simulink model "tres_tt_threeservos"  (Simulink 8.3)
settings: Solver=ode45  StartTime=0.0  StopTime=1.0  RelTol=1e-3
libraries: tres_simulink_blockset x4, truetime x1
settings Model: Creator=matteo  LastModifiedBy=matteo
settings OptimizationCC: ExpressionDepthLimit=2147483647
settings DebuggingCC: FcnCallInpInsideContextMsg=EnableAllAsWarning
settings GRTTargetCC: CombineOutputUpdateFcns=on  GRTInterface=off

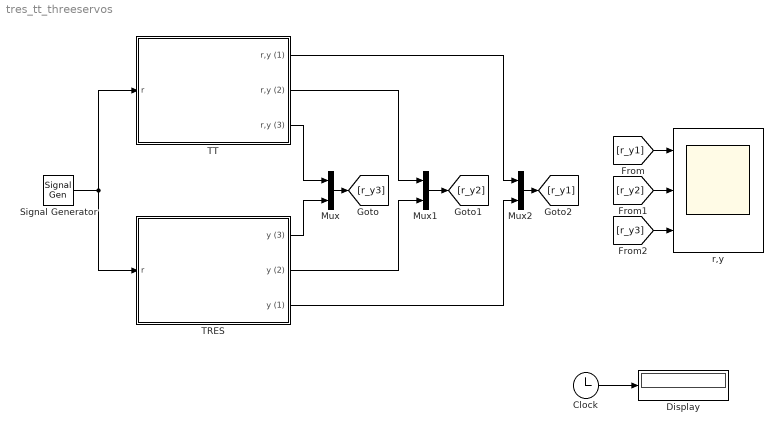
== system tres_tt_threeservos ==
  Clock : Clock
  Display : Display
  Mux : Mux  Inputs=2
  Mux1 : Mux  Inputs=2
  Mux2 : Mux  Inputs=2
  Signal Generator : SignalGenerator  WaveForm=square  Frequency=1.5
  TRES : Subsystem  TreatAsAtomicUnit=on
  TT : Subsystem  TreatAsAtomicUnit=on
  r,y : Scope  NumInputPorts=3
      settings: TimeRange=1  YMin=-2~-2~-2  YMax=2~2~2  SaveName=ry
  wires:
  Clock/1 -> Display/1
  TT/3(r,y (3)) -> Mux/1
  TRES/1(y (3)) -> Mux/2
  TRES/2(y (2)) -> Mux1/2
  TT/2(r,y (2)) -> Mux1/1
  TRES/3(y (1)) -> Mux2/2
  TT/1(r,y (1)) -> Mux2/1
  Mux/1 -> [r_y3]
  Mux1/1 -> [r_y2]
  Mux2/1 -> [r_y1]
  [r_y1] -> r,y/1
  [r_y2] -> r,y/2
  [r_y3] -> r,y/3
  Signal Generator/1 -> TT/1(r), TRES/1(r)

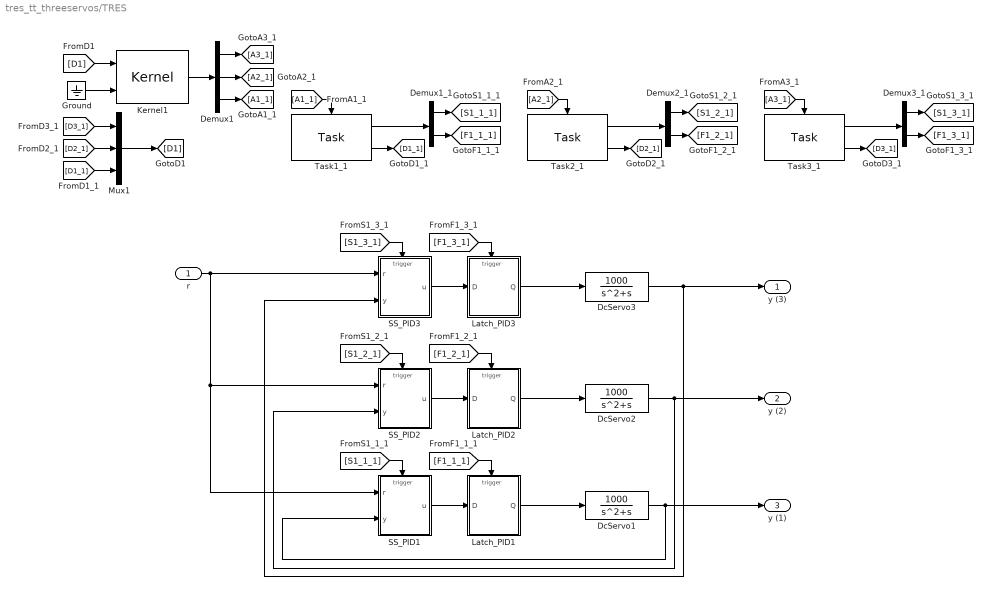
== system tres_tt_threeservos/TRES ==
  r : Inport
  DcServo1 : TransferFcn  Numerator=[1000]  Denominator=[1 1 0]
  DcServo2 : TransferFcn  Numerator=[1000]  Denominator=[1 1 0]
  DcServo3 : TransferFcn  Numerator=[1000]  Denominator=[1 1 0]
  Demux1 : Demux  Outputs=3
  Demux1_1 : Demux  Outputs=2
  Demux2_1 : Demux  Outputs=2
  Demux3_1 : Demux  Outputs=2
  Ground : Ground
  Kernel1 : tres_simulink_blockset/Kernel  taskset_descr_name=task_set_descr  scheduling_policy=DEADLINE_MONOTONIC  dead_miss_rule=Continue  time_res=Milli_Seconds  core_num=1  under_engine=RTSIM
  Latch_PID1 : Subsystem  TreatAsAtomicUnit=on
  Latch_PID2 : Subsystem  TreatAsAtomicUnit=on
  Latch_PID3 : Subsystem  TreatAsAtomicUnit=on
  Mux1 : Mux  Inputs=3
  SS_PID1 : Subsystem
  SS_PID2 : Subsystem
  SS_PID3 : Subsystem
  Task1_1 : tres_simulink_blockset/Task  conf_name=task1_1_descr
  Task2_1 : tres_simulink_blockset/Task  conf_name=task2_1_descr
  Task3_1 : tres_simulink_blockset/Task  conf_name=task3_1_descr
  y (3) : Outport
  y (2) : Outport  Port=2
  y (1) : Outport  Port=3
  wires:
  r/1 -> SS_PID1/1(r), SS_PID2/1(r), SS_PID3/1(r)
  DcServo3/1 -> SS_PID3/2(y), y (3)/1
  DcServo2/1 -> SS_PID2/2(y), y (2)/1
  DcServo1/1 -> SS_PID1/2(y), y (1)/1
  SS_PID3/1(u) -> Latch_PID3/1(D)
  SS_PID2/1(u) -> Latch_PID2/1(D)
  SS_PID1/1(u) -> Latch_PID1/1(D)
  Kernel1/1 -> Demux1/1
  Demux1/1 -> [A3_1]
  [D3_1] -> Mux1/1
  Demux1/2 -> [A2_1]
  [D2_1] -> Mux1/2
  Demux1/3 -> [A1_1]
  [D1_1] -> Mux1/3
  [D1] -> Kernel1/1
  Mux1/1 -> [D1]
  Task1_1/2 -> [D1_1]
  [A1_1] -> Task1_1/Trigger
  Task1_1/1 -> Demux1_1/1
  Demux1_1/1 -> [S1_1_1]
  Demux1_1/2 -> [F1_1_1]
  Task2_1/2 -> [D2_1]
  [A2_1] -> Task2_1/Trigger
  Task2_1/1 -> Demux2_1/1
  Demux2_1/1 -> [S1_2_1]
  Demux2_1/2 -> [F1_2_1]
  Task3_1/2 -> [D3_1]
  [A3_1] -> Task3_1/Trigger
  Task3_1/1 -> Demux3_1/1
  Demux3_1/1 -> [S1_3_1]
  Demux3_1/2 -> [F1_3_1]
  Latch_PID1/1(Q) -> DcServo1/1
  [S1_1_1] -> SS_PID1/Trigger
  [F1_1_1] -> Latch_PID1/Trigger
  Latch_PID2/1(Q) -> DcServo2/1
  [S1_2_1] -> SS_PID2/Trigger
  [F1_2_1] -> Latch_PID2/Trigger
  Latch_PID3/1(Q) -> DcServo3/1
  [S1_3_1] -> SS_PID3/Trigger
  [F1_3_1] -> Latch_PID3/Trigger
  Ground/1 -> Kernel1/2

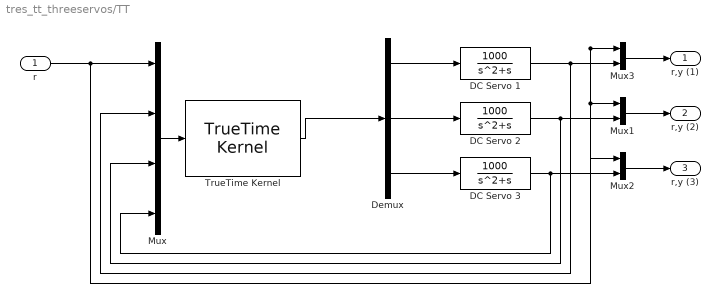
== system tres_tt_threeservos/TT ==
  r : Inport
  DC Servo 1 : TransferFcn  Numerator=[1000]  Denominator=[1 1 0]
  DC Servo 2 : TransferFcn  Numerator=[1000]  Denominator=[1 1 0]
  DC Servo 3 : TransferFcn  Numerator=[1000]  Denominator=[1 1 0]
  Demux : Demux  Outputs=3
  Mux : Mux
  Mux1 : Mux  Inputs=2
  Mux2 : Mux  Inputs=2
  Mux3 : Mux  Inputs=2
  TrueTime Kernel : truetime/TrueTime Kernel  sfun=tt_threeservos_init  args=1  ninputsoutputs=[4 3]  ntriggers=0  trigtype=falling  nwnodenbr=[]  clockoffsetdrift=[0 0]  schedoutput=off  battery=off  poweroutput=off
  r,y (1) : Outport
  r,y (2) : Outport  Port=2
  r,y (3) : Outport  Port=3
  wires:
  r/1 -> Mux1/1, Mux2/1, Mux3/1, Mux/1
  Demux/2 -> DC Servo 2/1
  Demux/3 -> DC Servo 3/1
  DC Servo 1/1 -> Mux3/2, Mux/2
  DC Servo 2/1 -> Mux1/2, Mux/3
  DC Servo 3/1 -> Mux2/2, Mux/4
  Mux2/1 -> r,y (3)/1
  Mux/1 -> TrueTime Kernel/1
  TrueTime Kernel/1 -> Demux/1
  Mux1/1 -> r,y (2)/1
  Mux3/1 -> r,y (1)/1
  Demux/1 -> DC Servo 1/1

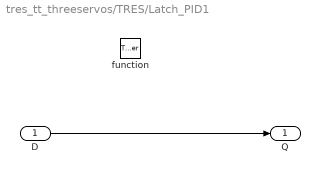
== system tres_tt_threeservos/TRES/Latch_PID1 ==
  D : Inport
  function : TriggerPort  TriggerType=function-call
  Q : Outport
  wires:
  D/1 -> Q/1

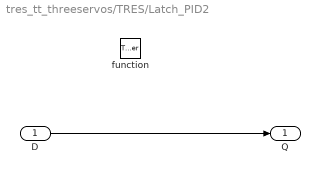
== system tres_tt_threeservos/TRES/Latch_PID2 ==
  D : Inport
  function : TriggerPort  TriggerType=function-call
  Q : Outport
  wires:
  D/1 -> Q/1

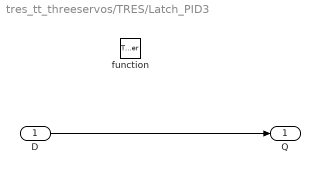
== system tres_tt_threeservos/TRES/Latch_PID3 ==
  D : Inport
  function : TriggerPort  TriggerType=function-call
  Q : Outport
  wires:
  D/1 -> Q/1

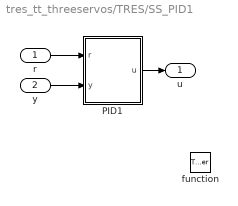
== system tres_tt_threeservos/TRES/SS_PID1 ==
  r : Inport
  y : Inport  Port=2
  function : TriggerPort  TriggerType=function-call
  PID1 : Subsystem  mask{K=0.96, Ti=0.12, Td=0.049, beta=0.5, N=10, h=0.006}
  u : Outport
  wires:
  r/1 -> PID1/1(r)
  y/1 -> PID1/2(y)
  PID1/1(u) -> u/1

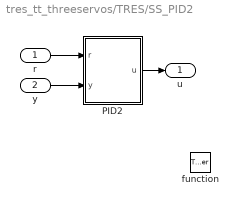
== system tres_tt_threeservos/TRES/SS_PID2 ==
  r : Inport
  y : Inport  Port=2
  function : TriggerPort  TriggerType=function-call
  PID2 : Subsystem  mask{K=0.96, Ti=0.12, Td=0.049, beta=0.5, N=10, h=0.005}
  u : Outport
  wires:
  r/1 -> PID2/1(r)
  y/1 -> PID2/2(y)
  PID2/1(u) -> u/1

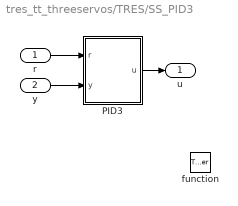
== system tres_tt_threeservos/TRES/SS_PID3 ==
  r : Inport
  y : Inport  Port=2
  function : TriggerPort  TriggerType=function-call
  PID3 : Subsystem  mask{K=0.96, Ti=0.12, Td=0.049, beta=0.5, N=10, h=0.004}
  u : Outport
  wires:
  r/1 -> PID3/1(r)
  y/1 -> PID3/2(y)
  PID3/1(u) -> u/1

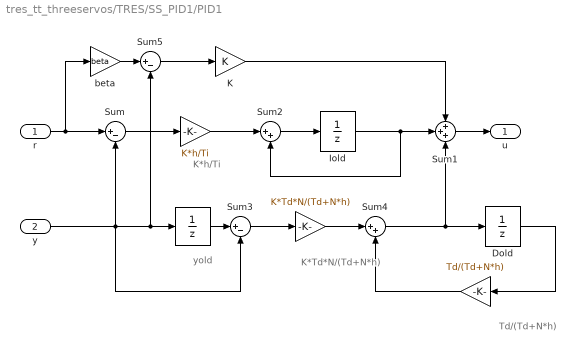
== system tres_tt_threeservos/TRES/SS_PID1/PID1 ==
  note: K*h/Ti
  note: K*Td*N/(Td+N*h)
  note: Td/(Td+N*h)
  note: yold
  r : Inport  SampleTime=-1.0
  y : Inport  Port=2  SampleTime=-1.0
  " " : UnitDelay  SampleTime=-1.0
  "   " : Gain  Gain=K*h/Ti  SampleTime=-1.0  SaturateOnIntegerOverflow=on  OutDataTypeStr=Inherit: Same as input  ParamDataTypeStr=Inherit: Same as input
  "             " : Gain  Gain=K*Td*N/(Td+N*h)  SampleTime=-1.0  SaturateOnIntegerOverflow=on  OutDataTypeStr=Inherit: Same as input  ParamDataTypeStr=Inherit: Same as input
  "              " : Gain  Gain=Td/(Td+N*h)  SampleTime=-1.0  SaturateOnIntegerOverflow=on  OutDataTypeStr=Inherit: Same as input  ParamDataTypeStr=Inherit: Same as input
  Dold : UnitDelay  SampleTime=-1.0
  "Iold " : UnitDelay  SampleTime=-1.0
  K : Gain  Gain=K  SampleTime=-1.0  SaturateOnIntegerOverflow=on  OutDataTypeStr=Inherit: Same as input  ParamDataTypeStr=Inherit: Same as input
  Sum : Sum  Inputs=|+-  SampleTime=-1.0  SaturateOnIntegerOverflow=on  InputSameDT=on  OutDataTypeStr=Inherit: Same as first input
  Sum1 : Sum  Inputs=+++  SampleTime=-1.0  SaturateOnIntegerOverflow=on  InputSameDT=on  OutDataTypeStr=Inherit: Same as first input
  Sum2 : Sum  Inputs=|++  SampleTime=-1.0  SaturateOnIntegerOverflow=on  InputSameDT=on  OutDataTypeStr=Inherit: Same as first input
  Sum3 : Sum  Inputs=|+-  SampleTime=-1.0  SaturateOnIntegerOverflow=on  InputSameDT=on  OutDataTypeStr=Inherit: Same as first input
  Sum4 : Sum  Inputs=|++  SampleTime=-1.0  SaturateOnIntegerOverflow=on  InputSameDT=on  OutDataTypeStr=Inherit: Same as first input
  Sum5 : Sum  Inputs=|+-  SampleTime=-1.0  SaturateOnIntegerOverflow=on  InputSameDT=on  OutDataTypeStr=Inherit: Same as first input
  beta : Gain  Gain=beta  SampleTime=-1.0  SaturateOnIntegerOverflow=on  OutDataTypeStr=Inherit: Same as input  ParamDataTypeStr=Inherit: Same as input
  u : Outport  SampleTime=-1.0
  wires:
  y/1 -> Sum/2, Sum3/2, " "/1, Sum5/2
  r/1 -> Sum/1, beta/1
  Sum1/1 -> u/1
  K/1 -> Sum1/1
  Sum2/1 -> "Iold "/1
  Dold/1 -> "              "/1
  "             "/1 -> Sum4/1
  Sum3/1 -> "             "/1
  Sum4/1 -> Dold/1, Sum1/3
  " "/1 -> Sum3/1
  "Iold "/1 -> Sum2/2, Sum1/2
  "   "/1 -> Sum2/1
  Sum/1 -> "   "/1
  "              "/1 -> Sum4/2
  beta/1 -> Sum5/1
  Sum5/1 -> K/1

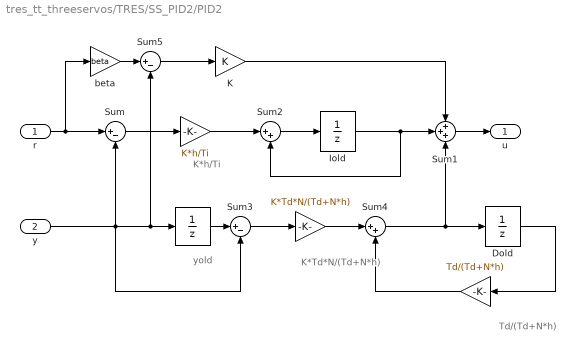
== system tres_tt_threeservos/TRES/SS_PID2/PID2 ==
  note: K*h/Ti
  note: K*Td*N/(Td+N*h)
  note: Td/(Td+N*h)
  note: yold
  r : Inport  SampleTime=-1.0
  y : Inport  Port=2  SampleTime=-1.0
  " " : UnitDelay  SampleTime=-1.0
  "   " : Gain  Gain=K*h/Ti  SampleTime=-1.0  SaturateOnIntegerOverflow=on  OutDataTypeStr=Inherit: Same as input  ParamDataTypeStr=Inherit: Same as input
  "             " : Gain  Gain=K*Td*N/(Td+N*h)  SampleTime=-1.0  SaturateOnIntegerOverflow=on  OutDataTypeStr=Inherit: Same as input  ParamDataTypeStr=Inherit: Same as input
  "              " : Gain  Gain=Td/(Td+N*h)  SampleTime=-1.0  SaturateOnIntegerOverflow=on  OutDataTypeStr=Inherit: Same as input  ParamDataTypeStr=Inherit: Same as input
  Dold : UnitDelay  SampleTime=-1.0
  "Iold " : UnitDelay  SampleTime=-1.0
  K : Gain  Gain=K  SampleTime=-1.0  SaturateOnIntegerOverflow=on  OutDataTypeStr=Inherit: Same as input  ParamDataTypeStr=Inherit: Same as input
  Sum : Sum  Inputs=|+-  SampleTime=-1.0  SaturateOnIntegerOverflow=on  InputSameDT=on  OutDataTypeStr=Inherit: Same as first input
  Sum1 : Sum  Inputs=+++  SampleTime=-1.0  SaturateOnIntegerOverflow=on  InputSameDT=on  OutDataTypeStr=Inherit: Same as first input
  Sum2 : Sum  Inputs=|++  SampleTime=-1.0  SaturateOnIntegerOverflow=on  InputSameDT=on  OutDataTypeStr=Inherit: Same as first input
  Sum3 : Sum  Inputs=|+-  SampleTime=-1.0  SaturateOnIntegerOverflow=on  InputSameDT=on  OutDataTypeStr=Inherit: Same as first input
  Sum4 : Sum  Inputs=|++  SampleTime=-1.0  SaturateOnIntegerOverflow=on  InputSameDT=on  OutDataTypeStr=Inherit: Same as first input
  Sum5 : Sum  Inputs=|+-  SampleTime=-1.0  SaturateOnIntegerOverflow=on  InputSameDT=on  OutDataTypeStr=Inherit: Same as first input
  beta : Gain  Gain=beta  SampleTime=-1.0  SaturateOnIntegerOverflow=on  OutDataTypeStr=Inherit: Same as input  ParamDataTypeStr=Inherit: Same as input
  u : Outport  SampleTime=-1.0
  wires:
  y/1 -> Sum/2, Sum3/2, " "/1, Sum5/2
  r/1 -> Sum/1, beta/1
  Sum1/1 -> u/1
  K/1 -> Sum1/1
  Sum2/1 -> "Iold "/1
  Dold/1 -> "              "/1
  "             "/1 -> Sum4/1
  Sum3/1 -> "             "/1
  Sum4/1 -> Dold/1, Sum1/3
  " "/1 -> Sum3/1
  "Iold "/1 -> Sum2/2, Sum1/2
  "   "/1 -> Sum2/1
  Sum/1 -> "   "/1
  "              "/1 -> Sum4/2
  beta/1 -> Sum5/1
  Sum5/1 -> K/1

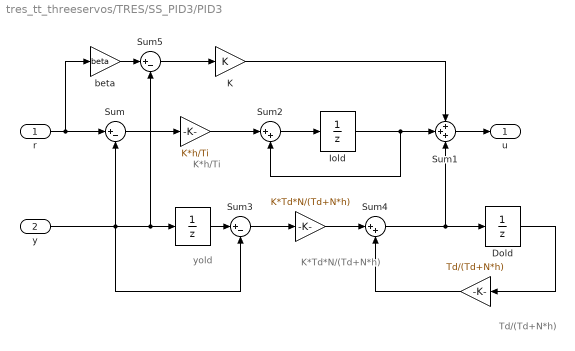
== system tres_tt_threeservos/TRES/SS_PID3/PID3 ==
  note: K*h/Ti
  note: K*Td*N/(Td+N*h)
  note: Td/(Td+N*h)
  note: yold
  r : Inport  SampleTime=-1.0
  y : Inport  Port=2  SampleTime=-1.0
  " " : UnitDelay  SampleTime=-1.0
  "   " : Gain  Gain=K*h/Ti  SampleTime=-1.0  SaturateOnIntegerOverflow=on  OutDataTypeStr=Inherit: Same as input  ParamDataTypeStr=Inherit: Same as input
  "             " : Gain  Gain=K*Td*N/(Td+N*h)  SampleTime=-1.0  SaturateOnIntegerOverflow=on  OutDataTypeStr=Inherit: Same as input  ParamDataTypeStr=Inherit: Same as input
  "              " : Gain  Gain=Td/(Td+N*h)  SampleTime=-1.0  SaturateOnIntegerOverflow=on  OutDataTypeStr=Inherit: Same as input  ParamDataTypeStr=Inherit: Same as input
  Dold : UnitDelay  SampleTime=-1.0
  "Iold " : UnitDelay  SampleTime=-1.0
  K : Gain  Gain=K  SampleTime=-1.0  SaturateOnIntegerOverflow=on  OutDataTypeStr=Inherit: Same as input  ParamDataTypeStr=Inherit: Same as input
  Sum : Sum  Inputs=|+-  SampleTime=-1.0  SaturateOnIntegerOverflow=on  InputSameDT=on  OutDataTypeStr=Inherit: Same as first input
  Sum1 : Sum  Inputs=+++  SampleTime=-1.0  SaturateOnIntegerOverflow=on  InputSameDT=on  OutDataTypeStr=Inherit: Same as first input
  Sum2 : Sum  Inputs=|++  SampleTime=-1.0  SaturateOnIntegerOverflow=on  InputSameDT=on  OutDataTypeStr=Inherit: Same as first input
  Sum3 : Sum  Inputs=|+-  SampleTime=-1.0  SaturateOnIntegerOverflow=on  InputSameDT=on  OutDataTypeStr=Inherit: Same as first input
  Sum4 : Sum  Inputs=|++  SampleTime=-1.0  SaturateOnIntegerOverflow=on  InputSameDT=on  OutDataTypeStr=Inherit: Same as first input
  Sum5 : Sum  Inputs=|+-  SampleTime=-1.0  SaturateOnIntegerOverflow=on  InputSameDT=on  OutDataTypeStr=Inherit: Same as first input
  beta : Gain  Gain=beta  SampleTime=-1.0  SaturateOnIntegerOverflow=on  OutDataTypeStr=Inherit: Same as input  ParamDataTypeStr=Inherit: Same as input
  u : Outport  SampleTime=-1.0
  wires:
  y/1 -> Sum/2, Sum3/2, " "/1, Sum5/2
  r/1 -> Sum/1, beta/1
  Sum1/1 -> u/1
  K/1 -> Sum1/1
  Sum2/1 -> "Iold "/1
  Dold/1 -> "              "/1
  "             "/1 -> Sum4/1
  Sum3/1 -> "             "/1
  Sum4/1 -> Dold/1, Sum1/3
  " "/1 -> Sum3/1
  "Iold "/1 -> Sum2/2, Sum1/2
  "   "/1 -> Sum2/1
  Sum/1 -> "   "/1
  "              "/1 -> Sum4/2
  beta/1 -> Sum5/1
  Sum5/1 -> K/1
